simulink library "root"  (R2024b)
settings: Solver=VariableStepAuto  StartTime=0.0  StopTime=10.0  RelTol=1e-3
libraries: config x1, notificaStato x1, luci x1, rgbled_temp x1
settings Model: Creator=mainuser  LastModifiedBy=mainuser

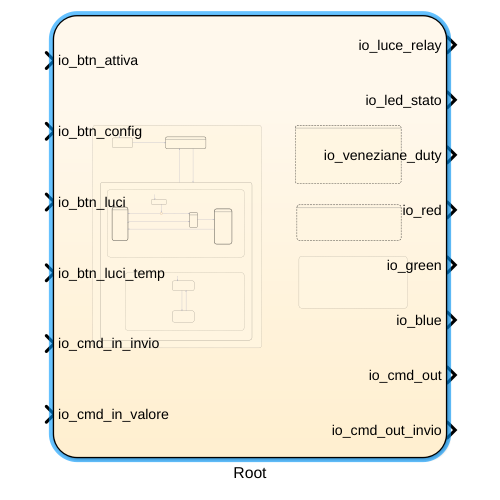
[thumbnail: Simulink's stored preview of the top-level diagram]
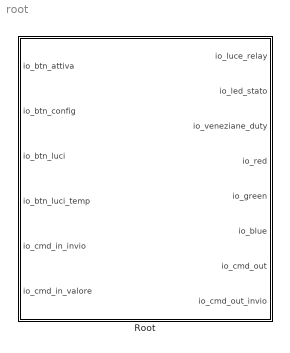
== system root ==
  Root : Stateflow chart  TreatAsAtomicUnit=on

== stateflow chart root/Root ==
  state Attivita [parallel]
    settings: executionOrder=1
    state Inattivo
      en:
      io_led_stato=false
      config_veneziane_gradi=0
      config_luci_sec=0
      ex_luci_state=config_luci_state;
      config_luci_state=false
      config_temp_rgb=16
    state Start
      config_is_valida=false
    state Atttivo
      state Attivo_Interfaccia [parallel]
        settings: executionOrder=1
        state Attivo_start
          config_luci_state=ex_luci_state;
        state Config
        state NotificaStato
        state AttivaNewconf
          config_veneziane_gradi=newconfig_veneziane_gradi
          config_luci_sec=newconfig_luci_sec
          config_temp_rgb=newconfig_temp_rgb
        (default) -> Attivo_start
        Attivo_start -> (junction 89)
        (junction 89) -> AttivaNewconf [order 2]
        (junction 89) -> Config [order 1] : [config_is_valida==false]
        AttivaNewconf -> NotificaStato
        145 -> AttivaNewconf : {config_is_valida=true}
        NotificaStato -> Config : [hasChangedTo(io_btn_config,true)]
      state Attivita_LED [parallel]
        settings: executionOrder=2
        state Attivo_ON
          en: io_led_stato=true;
        state Attivo_OFF
          en: io_led_stato=false;
        (default) -> Attivo_ON
        Attivo_ON -> Attivo_OFF : after(0.5,sec)
        Attivo_OFF -> Attivo_ON : after(0.5,sec)
    (default) -> Start
    Start -> Inattivo
    Atttivo -> Inattivo : [hasChangedTo(io_btn_attiva,true)]
    Inattivo -> Atttivo : [hasChangedTo(io_btn_attiva,true)]
  state Luci [parallel]
    settings: executionOrder=2
  state RGBLED_TEMP [parallel]
    settings: executionOrder=4
  state Veneziane [parallel]
    io_veneziane_duty = (double(config_veneziane_gradi) / 180) * 5 + 5;
    settings: executionOrder=3
  data: config_veneziane_gradi function_output; config_luci_sec function_output; config_temp function_output; config_luci_stato function_output; state_temp function_input; state_veneziane_gradi function_input; state_stato_luce function_input; config_temp_sec function_input; config_luce_state function_input; io_temp function_input; io_luce_relay output boolean size=1; config_is_valida local boolean size=1; newconfig_veneziane_gradi local uint8 size=1; config_veneziane_gradi local uint8 size=1; newconfig_luci_sec local uint8 size=1; config_luci_sec local uint8 size=1; newconfig_temp_rgb local uint8 size=1; config_temp_rgb local uint8 size=1; io_btn_attiva input boolean size=1; io_btn_config input boolean size=1; io_led_stato output boolean size=1; io_btn_luci input boolean size=1; io_btn_luci_temp input boolean size=1; io_cmd_in_invio input; io_cmd_in_valore input uint8; config_luci_state local boolean size=1; io_veneziane_duty output double; io_red output double size=1; io_green output double size=1; io_blue output double size=1; io_cmd_out output string; io_cmd_out_invio output boolean size=1; ex_luci_state local boolean size=1
